simulink model "HouseModelGeothermalHeater"  (R2022b)
settings: Solver=FixedStepAuto  StartTime=0.0  StopTime=4380  FixedStep=1  RelTol=1e-3  AbsTol=1e-6
model workspace (MATLAB code in the model file):
  | % load initial conditions and physical properties from file
  | 
  | sldemo_househeat_data
values from neighbouring files (symbols this model uses):
  c = 1005.4    [setVariables.m]
  M = (lenHouse*widHouse*htHouse+tan(pitRoof)*widHouse*lenHouse)*densAir    [setVariables.m]
  Mdot = 540    [setVariables.m]
  Req = RWall*RWindow/(RWall + RWindow)    [setVariables.m]
  THeater = 50    [setVariables.m]
  TinIC = 30    [setVariables.m]
libraries: simulink_extras x3
Description:
  | Thermal Model of a House
  | 
  | This demo illustrates how you can use Simulink(R) to create the thermal model of
  | a house. This system models the outdoor environment, the thermal
  | characteristics of the house, and the house heating system.
  | 
  | The sldemo_househeat_data.m file initializes data in the model workspace.
  | To make changes, you can edit the model workspace directly or edit the MATLAB(R) file
  | and re-load the model workspace.
  | 
  | To view the model workspace, select View > Model Explorer
  | from the Simulink editor.
  | 
  | Note: Time is given in units of hours
settings Model: Creator=The MathWorks, Inc.  LastModifiedBy=maazbhatti
settings SolverCC: AutoScaleAbsTol=off  AlgebraicLoopSolver=TrustRegion
settings DataIOCC: ExternalInput=[]  InitialState=[]  SaveFormat=Array  SaveOutput=off  SaveTime=off  SignalLoggingName=sldemo_househeat_output
settings OptimizationCC: BlockReduction=off  BooleanDataType=off  ExpressionDepthLimit=2147483647  InitFltsAndDblsToZero=on  LifeSpan=inf  BufferReusableBoundary=off
settings DebuggingCC: SaveWithParameterizedLinksMsg=none  UnderspecifiedInitializationDetection=Classic  MergeDetectMultiDrivingBlocksExec=none  SignalResolutionControl=TryResolveAllWithWarning  MultiTaskDSMMsg=warning  MultiTaskCondExecSysMsg=none  IntegerOverflowMsg=none  FcnCallInpInsideContextMsg=warning  UnconnectedInputMsg=warning  UnconnectedOutputMsg=warning  UnconnectedLineMsg=warning  BusObjectLabelMismatch=none  StateNameClashWarn=warning  SFUnexpectedBacktrackingDiag=warning  SFNoUnconditionalDefaultTransitionDiag=warning  SFExecutionAtInitializationDiag=none  SFMachineParentedDataDiag=warning  IntegerSaturationMsg=none  ArithmeticOperatorsInVariantConditions=warning
settings HardwareCC: ProdBitPerPointer=32  ProdBitPerSizeT=32  ProdBitPerPtrDiffT=32  ProdLargestAtomicFloat=None  ProdIntDivRoundTo=Undefined  ProdEndianess=Unspecified  ProdWordSize=32  ProdHWDeviceType=32-bit Generic  TargetUnknown=on
settings ModelReferenceCC: EnableRefExpFcnMdlSchedulingChecks=on  PropagateSignalLabelsOutOfModel=off
settings SFSimCC: SimUseLocalCustomCode=off  CustomCodeUndefinedFunction=UseInterfaceOnly
settings RTWCC: RTWUseLocalCustomCode=off
settings CodeAppCC: StateflowObjectComments=on
settings GRTTargetCC: TargetFcnLib=ansi_tfl_tmw.mat  TargetLangStandard=C89/C90 (ANSI)  CombineOutputUpdateFcns=off  GRTInterface=on
settings ConfigComp: CovMetricSettings=dw  CovSaveCumulativeToWorkspaceVar=on  CovSaveSingleToWorkspaceVar=on  CovExternalEMLEnable=off

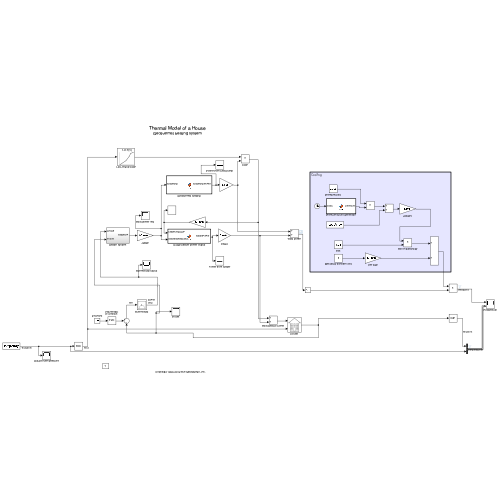
[thumbnail: Simulink's stored preview of the top-level diagram]
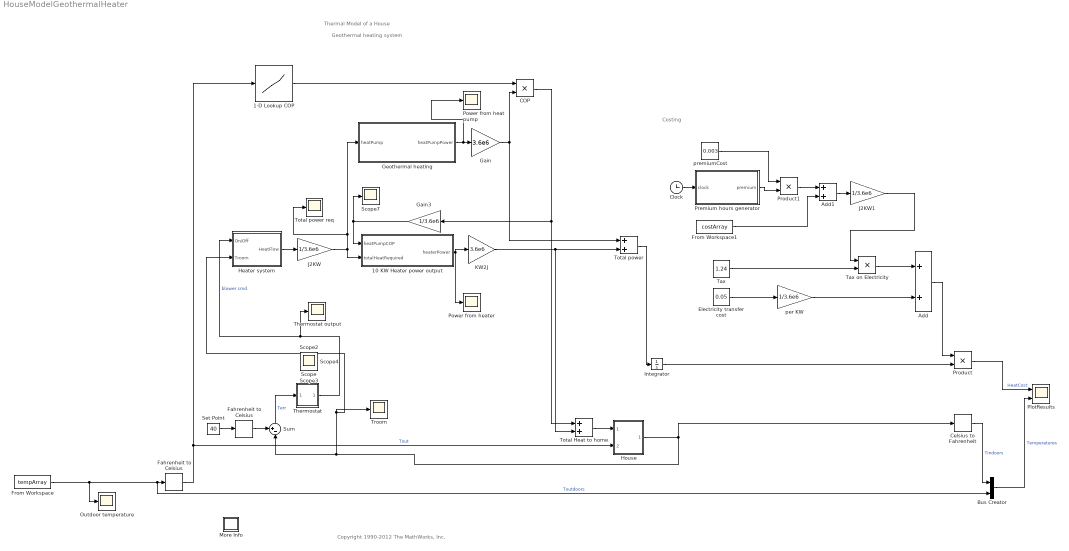
== system HouseModelGeothermalHeater ==
  note: Copyright 1990-2012 The MathWorks, Inc.
  note: Thermal Model of a House
  note: Geothermal heating system
  note: Costing
  1-D Lookup COP : Lookup_n-D  NumberOfTableDimensions=1  BreakpointsForDimension1=[-25,-7,2,7,12,15]  Table=[2,3,4.1,4.9,5,5.1]  InternalRulePriority=Speed  RndMeth=Simplest
  10 KW Heater power output : MATLAB Function  TreatAsAtomicUnit=on
  Add : Sum
  Add1 : Sum
  Bus Creator : BusCreator  Inputs=2
  COP : Product
  Celsius to Fahrenheit : simulink_extras/Transformations/Celsius to Fahrenheit
  Clock : Clock
  Electricity transfer cost : Constant  Value=0.05
  Fahrenheit to Celsius : simulink_extras/Transformations/Fahrenheit to Celsius
  "Fahrenheit to Celsius " : simulink_extras/Transformations/Fahrenheit to Celsius
  From Workspace : FromWorkspace  VariableName=tempArray
  From Workspace1 : FromWorkspace  VariableName=costArray
  Gain : Gain  Gain=3.6e6
  Gain3 : Gain  Gain=1/3.6e6
  Geothermal heating : MATLAB Function  TreatAsAtomicUnit=on
  Heater system : Subsystem
  House : Subsystem
      mask Display: image(fullfile(matlabroot,'toolbox','simulink','simdemos','simgeneral','images','HouseHeatHousePix.svg'))
  Integrator : Integrator
  J2KW : Gain  Gain=1/3.6e6
  J2KW1 : Gain  Gain=1/3.6e6
  KW2J : Gain  Gain=3.6e6
  More Info : Subsystem
      settings: OpenFcn=showExample('simulink_general/sldemo_househeatExample')
      mask Display: disp('?')
  Outdoor temperature : Scope
  PlotResults : Scope  NumInputPorts=2
  Power from heat pump : Scope
  Power from heater : Scope
  Premium hours generator : MATLAB Function  TreatAsAtomicUnit=on
  Product : Product
  Product1 : Product
  Scope{,2..4,7} (5 alike) : Scope
  Set Point : Constant  Value=40
  Sum : Sum  Inputs=+-|  InputSameDT=on  SaturateOnIntegerOverflow=on  OutDataTypeStr=Inherit: Same as first input
  Tax : Constant  Value=1.24  SampleTime=-1
  Tax on Electricity : Product
  Thermostat : Subsystem
      mask Display: image(fullfile(matlabroot,'toolbox','simulink','simdemos','simgeneral','images','HouseHeatThermostatPix.svg'))
  Thermostat output : Scope
  Total Heat to home : Sum
  Total power : Sum
  Total power req : Scope
  Troom : Scope
  per KW : Gain  Gain=1/3.6e6
  premiumCost : Constant  Value=0.003
  wires:
  Integrator/1 -> Product/2
  Thermostat/1(Blower switch) -> Thermostat output/1, Heater system/1(On/Off)  "blower cmd"
  Sum/1 -> Thermostat/1(Terr)  "Terr"
  House/1(Room Temp Troom) -> Sum/2, Troom/1, Heater system/2(Troom), Celsius to Fahrenheit/1
  Celsius to Fahrenheit/1 -> Bus Creator/1  "Tindoors"
  Fahrenheit to Celsius/1 -> 1-D Lookup COP/1, House/2(Outdoor Temp Tout)  "Tout"
  Bus Creator/1 -> PlotResults/2  "Temperatures"
  Product/1 -> PlotResults/1  "HeatCost"
  "Fahrenheit to Celsius "/1 -> Sum/1
  Set Point/1 -> "Fahrenheit to Celsius "/1
  Heater system/1(HeatFlow) -> J2KW/1
  Total Heat to home/1 -> House/1(Heater QDot In)
  J2KW/1 -> 10 KW Heater power output/2(totalHeatRequired), Geothermal heating/1(heatPump), Total power req/1
  Total power/1 -> Integrator/1
  1-D Lookup COP/1 -> COP/1
  Geothermal heating/1(heatPumpPower) -> Power from heat pump/1, Gain/1
  Gain/1 -> Total power/1, COP/2
  COP/1 -> Total Heat to home/1, Gain3/1
  10 KW Heater power output/1(heaterPower) -> KW2J/1, Power from heater/1
  KW2J/1 -> Total Heat to home/2, Total power/2
  Gain3/1 -> 10 KW Heater power output/1(heatPumpCOP), Scope7/1
  From Workspace/1 -> Outdoor temperature/1, Bus Creator/2, Fahrenheit to Celsius/1  "Toutdoors"
  Clock/1 -> Premium hours generator/1(clock)
  Tax/1 -> Tax on Electricity/2
  Tax on Electricity/1 -> Add/1
  Electricity transfer cost/1 -> per KW/1
  J2KW1/1 -> Tax on Electricity/1
  per KW/1 -> Add/2
  Product1/1 -> Add1/1
  Add1/1 -> J2KW1/1
  Premium hours generator/1(premium) -> Product1/2
  premiumCost/1 -> Product1/1
  From Workspace1/1 -> Add1/2
  Add/1 -> Product/1

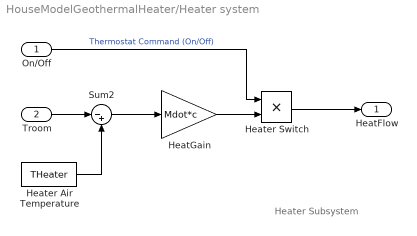
== system HouseModelGeothermalHeater/Heater system ==
  note: Heater Subsystem
  On/Off : Inport
  Troom : Inport  Port=2
  HeatGain : Gain  Gain=Mdot*c
  Heater Air Temperature : Constant  Value=THeater
  Heater Switch : Product  RndMeth=Zero
  Sum2 : Sum  Inputs=|-+
  HeatFlow : Outport  VectorParamsAs1DForOutWhenUnconnected=off
  wires:
  Heater Air Temperature/1 -> Sum2/2
  Troom/1 -> Sum2/1
  Sum2/1 -> HeatGain/1
  On/Off/1 -> Heater Switch/1  "Thermostat Command (On/Off)"
  HeatGain/1 -> Heater Switch/2
  Heater Switch/1 -> HeatFlow/1

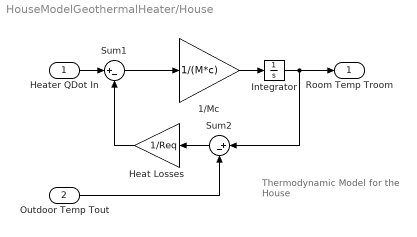
== system HouseModelGeothermalHeater/House ==
  note: Thermodynamic Model
      | for the House
  Heater QDot In : Inport
  Outdoor Temp Tout : Inport  Port=2
  1/Mc : Gain  Gain=1/(M*c)  SaturateOnIntegerOverflow=on  OutDataTypeStr=Inherit: Same as input  ParamDataTypeStr=Inherit: Same as input
  Heat Losses : Gain  Gain=1/Req  SaturateOnIntegerOverflow=on  OutDataTypeStr=Inherit: Same as input  ParamDataTypeStr=Inherit: Same as input
  Integrator : Integrator  InitialCondition=TinIC
  Sum1 : Sum  Inputs=|+-  InputSameDT=on  SaturateOnIntegerOverflow=on  OutDataTypeStr=Inherit: Same as first input
  Sum2 : Sum  Inputs=|+-  InputSameDT=on  SaturateOnIntegerOverflow=on  OutDataTypeStr=Inherit: Same as first input
  Room Temp Troom : Outport  InitialOutput=0  VectorParamsAs1DForOutWhenUnconnected=off
  wires:
  Outdoor Temp Tout/1 -> Sum2/2
  Heater QDot In/1 -> Sum1/1
  Sum1/1 -> 1/Mc/1
  Sum2/1 -> Heat Losses/1
  Heat Losses/1 -> Sum1/2
  1/Mc/1 -> Integrator/1
  Integrator/1 -> Sum2/1, Room Temp Troom/1

== system HouseModelGeothermalHeater/More Info ==

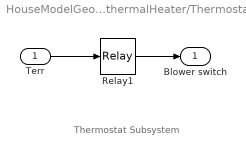
== system HouseModelGeothermalHeater/Thermostat ==
  note: Thermostat Subsystem
  Terr : Inport
  Relay1 : Relay  OnSwitchValue=5*(5/9)  OffSwitchValue=-5*(5/9)
  Blower switch : Outport  InitialOutput=0  VectorParamsAs1DForOutWhenUnconnected=off
  wires:
  Terr/1 -> Relay1/1
  Relay1/1 -> Blower switch/1

== matlab function HouseModelGeothermalHeater/Geothermal heating ==
  data: heatPump input; heatPumpPower output
function heatPumpPower = fcn(heatPump)
%Max power of geothermal heater
maxPower = 12;
heatPumpPower = heatPump;

%Assure that the heat pump does not exceed power of 5.5 KW
if (heatPump > maxPower)
    heatPumpPower = maxPower;
end

== matlab function HouseModelGeothermalHeater/Premium hours generator ==
  data: clock input; premium output
function premium = fcn(clock)

%Every other hour is assumed to be premium
premium = mod(clock,2);

end

== matlab function HouseModelGeothermalHeater/10 KW Heater power output ==
  data: heatPumpCOP input; totalHeatRequired input; heaterPower output
function heaterPower = fcn(heatPumpCOP, totalHeatRequired)

%If heat output from heat pump after COP is enough to warm the house then 10 KW heater is not
%required. Else it is
if(heatPumpCOP>=totalHeatRequired)
    heaterPower = 0;
else
    heaterPower = abs(totalHeatRequired-heatPumpCOP);
    if heaterPower > 10
        heaterPower = 10;
    end
end
